simulink library "Storage_Type_3"  (R2018b)
settings: Solver=ode45  StartTime=0.0  StopTime=10.0  RelTol=1e-3  EnableMultiTasking=on
undefined symbols (not defined in the file): path_carnot
libraries: carnot x10
settings Model: Creator=bernd.hafner  LastModifiedBy=drhf
settings DataIOCC: LimitDataPoints=on  SaveFormat=Array  SignalLoggingSaveFormat=ModelDataLogs
settings OptimizationCC: ExpressionDepthLimit=2147483647  LifeSpan=inf
settings DebuggingCC: UnderspecifiedInitializationDetection=Classic  MergeDetectMultiDrivingBlocksExec=none  SolverPrmCheckMsg=warning  FcnCallInpInsideContextMsg=warning  StateNameClashWarn=warning  SFUnexpectedBacktrackingDiag=warning  SFNoUnconditionalDefaultTransitionDiag=warning  SFExecutionAtInitializationDiag=none
settings HardwareCC: ProdBitPerPointer=32  ProdBitPerSizeT=32  ProdBitPerPtrDiffT=32  ProdLargestAtomicFloat=None  ProdIntDivRoundTo=Undefined  ProdEndianess=Unspecified  ProdWordSize=32  ProdHWDeviceType=32-bit Generic
settings ModelReferenceCC: PropagateSignalLabelsOutOfModel=off
settings SFSimCC: SimUseLocalCustomCode=off
settings RTWCC: RTWUseLocalCustomCode=off
settings CodeAppCC: StateflowObjectComments=on
settings GRTTargetCC: TargetLangStandard=C89/C90 (ANSI)  CombineOutputUpdateFcns=off  GRTInterface=on
settings ConfigComp: CovMetricSettings=dw  CovHtmlReporting=on  CovSaveCumulativeToWorkspaceVar=on  CovSaveSingleToWorkspaceVar=on  CovExternalEMLEnable=off

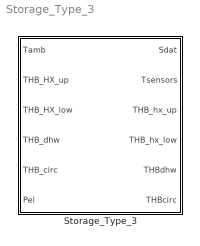
== system Storage_Type_3 ==
  Storage_Type_3 : Subsystem  mask(Storage for solar assisted hot water production){t0=[10:5:55], hgt=1.7684, stgtype=3, tini=[10 15 20 25 30 35 40 45 50 55], mpts=[1 2 3 4 5 6 7 8 9 10], PathName=fullfile(path_carnot('libsl'), 'Storage', 'Thermal', 'Storage_Type_3', 'parameter_set'), FileName='StorageType3_400_L.mat', userPath=off, userParam=off, uwall=1, ubot=1, utop=1, axcond=1, volume=0.5, dia=0.6, standing=standing cylinder, nodes=10, mpoints=10, Tsensor=[0.1 0.5 0.7], hx1inlet=0.8, hx1outlet=0.6, hx1dia=0.03, hx1uac=50, hx1uam=0.15, hx1uat=0.6, hx1_uat2=0, hx1dpqua=20, hx1dplin=20, hx2inlet=0.4, hx2outlet=0, hx2dia=0.03, hx2uac=100, hx2uam=0.15, hx2uat=0.6, hx2_uat2=0, hx2dplin=30, hx2dpqua=30, pipe1inlet=0, pipe1outlet=1, pipe1dia=0.03, pipe2inlet=0.6, pipe2outlet=1, pipe2dia=0.03, heater1start=0.6, heater1end=0.65}
      mask prompts: t0 "Initial temperature (vector or scalar) in °C"; hgt "Height of storage in m"; stgtype "Storage Type (0..5)"; tini "Start temperatures of nodes in °C"; mpts "Index to measured nodes"; PathName "Path"; FileName "Parameter set"; userPath "Edit path and name of parameter set"; userParam "User defined parameters"; uwall "Heat transfer coefficient to ambient [W/m²K]"; ubot "Heat transfer coefficient to ambient bottom [W/m²K]"; utop "Heat transfer coefficient to ambient top [W/m²K]"; axcond "Effective thermal conductivity [W/m/K]"; volume "Volume [m³]"; dia "Diameter [m]"; standing "Position"; nodes "Number of nodes"; mpoints "Number of node temperatures (for display)"; Tsensor "Temperature sensor position (0..1, 0 = bottom, 1 = top)"; hx1inlet "relative height of inlet"; hx1outlet "relative height of outlet"; hx1dia "Diameter of HX pipe [m]"; hx1uac "uac: heat transfer coefficient [W/K /(kg/s) /(°C)]"; hx1uam "uam: massflow dependent heat transfer [-]"; hx1uat "uat: temperature dependent heat transfer [-]"; hx1_uat2 "uat2: temperature difference dependent heat transfer [-]"; hx1dpqua "pressure drop quadratic in mdot [Pa*s²/kg²]"; hx1dplin "pressure drop linear in mdot [Pa*s/kg]"; hx2inlet "relative height of inlet"; hx2outlet "relative height of outlet"; hx2dia "Diameter of HX pipe [m]"; hx2uac "uac: heat transfer coefficient [W/K /(kg/s) /(°C)]"; hx2uam "uam: massflow dependent heat transfer [-]"; hx2uat "uat: temperature dependent heat transfer [-]"; hx2_uat2 "uat2: temperature difference dependent heat transfer [-]"; hx2dplin "pressure drop linear in mdot [Pa*s/kg]"; hx2dpqua "pressure drop quadratic in mdot [Pa*s²/kg²]"; pipe1inlet "relative height of inlet, range from 0 (= bottom) to 1 (= top)"; pipe1outlet "relative height of outlet, range from 0 (= bottom) to 1 (= top)"; pipe1dia "Diameter of pipe in m"; pipe2inlet "relative height of inlet, range from 0 (= bottom) to 1 (= top)"; pipe2outlet "relative height of outlet, range from 0 (= bottom) to 1 (= top)"; pipe2dia "Diameter of pipe in m"; heater1start "relative height start heating zone"; heater1end "relative height end heating zone"
      mask help:
      | Storage for hot water production (domestic hot water cylinder) with two heat exchangers.
      | The storage model has the following components (with their typical position):
      | - one solar heat exchanger (lower part)
      | - one backup heater heat exchanger (upper part)
      | - one pipe connection for the domestic hot water (total height)
      | - one pipe connection hot water circulation (upper part )
      mask init:
      | [ok, param] = CarnotCallbacks_StorageConf('SetParam',stgtype,gcbh,PathName,FileName);
      mask Help: web(fullfile(path_carnot('help'),'Storage_Type_N.html'),'-helpbrowser')
      mask TypeOptions hgt: HX_EN12977_1/hgt | HX_EN12977_2/hgt | Pipe_Connection_1/hgt | Pipe_Connection_2/hgt
      mask TypeOptions stgtype: CreateSdat/stgtype
      mask TypeOptions tini: sfun_storageTnodes/tini
      mask TypeOptions mpts: select_T/Indices
      mask Callback userPath: [ok, param] = CarnotCallbacks_StorageConf('UserEdit',3,gcbh);
      mask Callback userParam: [ok, param] = CarnotCallbacks_StorageConf('UserEdit',3,gcbh);
      mask TypeOptions uwall: sfun_storageTnodes/uloss
      mask TypeOptions ubot: sfun_storageTnodes/ubot
      mask TypeOptions utop: sfun_storageTnodes/utop
      mask TypeOptions axcond: sfun_storageTnodes/cond
      mask TypeOptions volume: sfun_storageTnodes/volume | CreateSdat/volume
      mask TypeOptions dia: sfun_storageTnodes/dia | Pipe_Connection_1/dstg | Pipe_Connection_2/dstg
      mask TypeOptions standing: sfun_storageTnodes/standing
      mask TypeOptions nodes: sfun_storageTnodes/nodes | select_T/InputPortWidth | HX_EN12977_1/nodes | HX_EN12977_2/nodes | Pipe_Connection_1/nodes | Pipe_Connection_2/nodes
      mask TypeOptions Tsensor: T_Sensor_Surface/pos
      mask TypeOptions hx1inlet: HX_EN12977_1/h_in
      mask TypeOptions hx1outlet: HX_EN12977_1/h_out
      mask TypeOptions hx1dia: HX_EN12977_1/dia
      mask TypeOptions hx1uac: HX_EN12977_1/ua0
      mask TypeOptions hx1uam: HX_EN12977_1/uam
      mask TypeOptions hx1uat: HX_EN12977_1/uat
      mask TypeOptions hx1_uat2: HX_EN12977_1/uat2
      mask TypeOptions hx1dpqua: HX_EN12977_1/dpqua
      mask TypeOptions hx1dplin: HX_EN12977_1/dplin
      mask TypeOptions hx2inlet: HX_EN12977_2/h_in
      mask TypeOptions hx2outlet: HX_EN12977_2/h_out
      mask TypeOptions hx2dia: HX_EN12977_2/dia
      mask TypeOptions hx2uac: HX_EN12977_2/ua0
      mask TypeOptions hx2uam: HX_EN12977_2/uam
      mask TypeOptions hx2uat: HX_EN12977_2/uat
      mask TypeOptions hx2_uat2: HX_EN12977_2/uat2
      mask TypeOptions hx2dplin: HX_EN12977_2/dplin
      mask TypeOptions hx2dpqua: HX_EN12977_2/dpqua
      mask TypeOptions pipe1inlet: Pipe_Connection_1/h_in
      mask TypeOptions pipe1outlet: Pipe_Connection_1/h_out
      mask TypeOptions pipe1dia: Pipe_Connection_1/dpipe
      mask TypeOptions pipe2inlet: Pipe_Connection_2/h_in
      mask TypeOptions pipe2outlet: Pipe_Connection_2/h_out
      mask TypeOptions pipe2dia: Pipe_Connection_2/dpipe
      mask TypeOptions heater1start: Electric_Heating_1/hin
      mask TypeOptions heater1end: Electric_Heating_1/hout
      mask DialogControl Container14 Prompt: Infos
      mask DialogControl ParameterGroupVar Prompt: Picking a parameter set
      mask DialogControl Control3 Prompt: Carnot public data
      mask DialogControl Control3 Callback: [ok, file] = CarnotCallbacks_StorageConf('GetFilename',3,gcbh,'public');
      mask DialogControl Control4 Prompt: Carnot internal data
      mask DialogControl Control4 Callback: [ok, file] = CarnotCallbacks_StorageConf('GetFilename',3,gcbh,'internal');
      mask DialogControl Control2 Prompt: Selected path
      mask DialogControl Control2 Callback: [ok, file] = CarnotCallbacks_StorageConf('GetFilename',3,gcbh,'selected');
      mask DialogControl Container4 Prompt: Parameter values
      mask DialogControl Container6 Prompt: Storage
      mask DialogControl Container8 Prompt: Connections
      mask DialogControl Container11 Prompt: Upper heat exchanger
      mask DialogControl Container13 Prompt: Lower heat exchanger
      mask DialogControl Container9 Prompt: Discharging pipe
      mask DialogControl Container12 Prompt: Circulation pipe
      mask DialogControl Container17 Prompt: Electric Heating
      mask DialogControl Container20 Prompt: Heater 1
      mask DialogControl Control6 Prompt: Save in Carnot internal data
      mask DialogControl Control6 Callback: [ok, param] = CarnotCallbacks_StorageConf('SaveFilename',3,gcbh,'internal','STG');
      mask DialogControl Control5 Prompt: Save in selected path
      mask DialogControl Control5 Callback: [ok, param] = CarnotCallbacks_StorageConf('SaveFilename',3,gcbh,'selected','STG');
      mask Display:
      | % user defined picture file
      | namestr = ['Storage_Type_', num2str(get_param(gcb,'stgtype'))];
      | picfile = fullfile(path_carnot('intlibsl'), 'Storage','Thermal', ...
      |     namestr,'parameter_set', [namestr, '.jpg']);
      | 
      | % show internal picture if defined
      | pic = false;
      | if  ~BlockIsInCarnotLibrary       % if not located in library
      |     if exist(picfile, 'file')
      |         image(imread(picfile), [0.25, 0, 0.45, 1])
      |         set_param(gcb, 'BackgroundColor', 'White')
      |         pic = true;
      |     end
      | end
      | 
      | % show public picture
      | if ~pic
      |     set_param(gcb, 'BackgroundColor', 'Red')
      |     plot([36,36,40,50,54,54,50,40,36]/90,[90,50,45,45,50,90,93,93,90]/100, ...
      |         [36,51,40,51,36]/90,[77,77,81,85,85]/100,[36,51,44,51,36]/90, ...
      |         [50,50,55,60,60]/100,...
      |         [36,50,50,36]/90,[75,75,74,74]/100,...
      |         [36,34,34,36]/90,[76.5,76.5,73,73]/100)
      | end

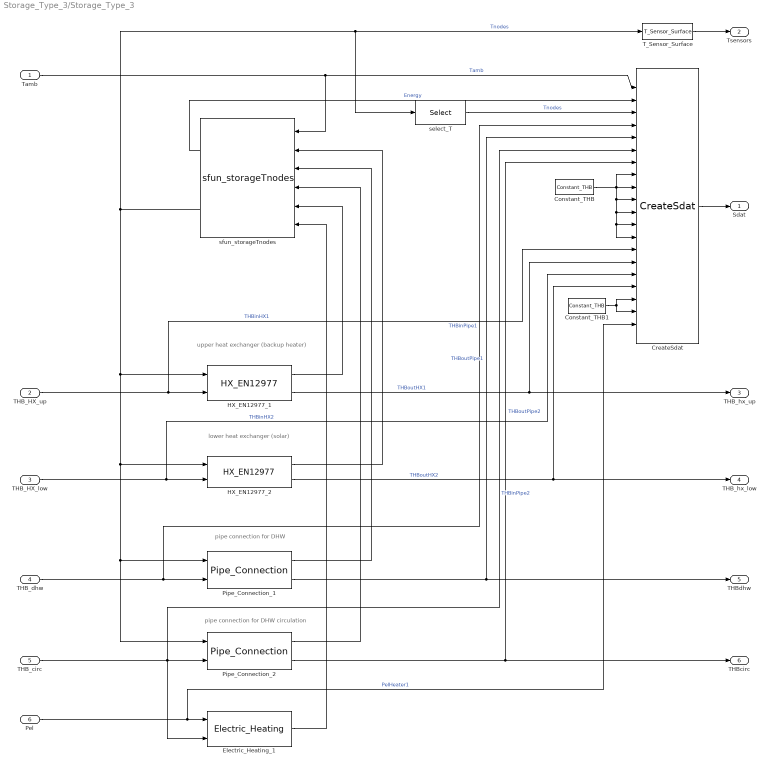
== system Storage_Type_3/Storage_Type_3 ==
  note: upper heat exchanger (backup heater)
  note: pipe connection for DHW
  note: pipe connection for DHW circulation
  note: lower heat exchanger (solar)
  Tamb : Inport
  THB_HX_up : Inport  Port=2
  THB_HX_low : Inport  Port=3
  THB_dhw : Inport  Port=4
  THB_circ : Inport  Port=5
  Pel : Inport  Port=6
  Constant_THB : carnot/Source/Simple/Constant_THB  t=20  mdot=0  p=1e5  mID=No Pressure Drop  fluid=Water  mix=0  mix2=0  mix3=0  dia=0.02  hgt=0
      settings: SourceProductName=Carnot
  Constant_THB1 : carnot/Source/Simple/Constant_THB  t=20  mdot=0  p=1e5  mID=No Pressure Drop  fluid=Water  mix=0  mix2=0  mix3=0  dia=0.02  hgt=0
      settings: SourceProductName=Carnot
  CreateSdat : carnot/Basic/Thermal_Models/CreateSdat  volume=volume  stgtype=stgtype
      settings: SourceProductName=Carnot
  Electric_Heating_1 : carnot/Storage/Thermal/Storage_Ports/Electric_Heating  hin=heater1start  hout=heater1end  nodes=nodes
      settings: SourceProductName=Carnot
  HX_EN12977_1 : carnot/Storage/Thermal/Storage_Ports/HX_EN12977  h_in=hx1inlet  h_out=hx1outlet  hgt=hgt  dia=hx1dia  height=-0.35368  ua0=hx1uac  uam=hx1uam  uat=hx1uat  uat2=hx1_uat2  dplin=hx1dplin  dpqua=hx1dpqua  nodes=nodes
      settings: SourceProductName=Carnot
  HX_EN12977_2 : carnot/Storage/Thermal/Storage_Ports/HX_EN12977  h_in=hx2inlet  h_out=hx2outlet  hgt=hgt  dia=hx2dia  height=-0.70736  ua0=hx2uac  uam=hx2uam  uat=hx2uat  uat2=hx2_uat2  dplin=hx2dplin  dpqua=hx2dpqua  nodes=nodes
      settings: SourceProductName=Carnot
  Pipe_Connection_1 : carnot/Storage/Thermal/Storage_Ports/Pipe_Connection  h_in=pipe1inlet  h_out=pipe1outlet  hgt=hgt  dpipe=pipe1dia  dstg=dia  height=1.7684  nodes=nodes
      settings: SourceProductName=Carnot
  Pipe_Connection_2 : carnot/Storage/Thermal/Storage_Ports/Pipe_Connection  h_in=pipe2inlet  h_out=pipe2outlet  hgt=hgt  dpipe=pipe2dia  dstg=dia  height=0.70736  nodes=nodes
      settings: SourceProductName=Carnot
  T_Sensor_Surface : carnot/Control/T_Sensor_Surface  pos=Tsensor  tdel=10  t0=mean(tini)
      settings: SourceProductName=Carnot
  select_T : Selector  InputPortWidth=nodes  IndexOptions=Index vector (dialog)  Indices=[1 2 3 4 5 6 7 8 9 10]  OutputSizes=1
  sfun_storageTnodes : carnot/Basic/Thermal_Models/sfun_storageTnodes  uloss=uwall  ubot=ubot  utop=utop  cond=axcond  volume=volume  dia=dia  standing=standing cylinder  tini=tini  nodes=nodes  nconnect=5  elimthermocline=2  condinvtc=1e5
      settings: SourceProductName=Carnot
  Sdat : Outport
  Tsensors : Outport  Port=2
  THB_hx_up : Outport  Port=3
  THB_hx_low : Outport  Port=4
  THBdhw : Outport  Port=5
  THBcirc : Outport  Port=6
  wires:
  Constant_THB/1 -> CreateSdat/9, CreateSdat/8, CreateSdat/13, CreateSdat/12, CreateSdat/11, CreateSdat/10
  Constant_THB1/1 -> CreateSdat/19, CreateSdat/18
  sfun_storageTnodes/1 -> CreateSdat/2  "Energy"
  HX_EN12977_1/1 -> sfun_storageTnodes/5
  Pipe_Connection_2/2 -> CreateSdat/7, THBcirc/1  "THBoutPipe2"
  Pipe_Connection_2/1 -> sfun_storageTnodes/4
  THB_circ/1 -> Electric_Heating_1/2, Pipe_Connection_2/2, CreateSdat/6  "THBinPipe2"
  Tamb/1 -> CreateSdat/1, sfun_storageTnodes/1  "Tamb"
  THB_HX_low/1 -> HX_EN12977_2/2, CreateSdat/16  "THBinHX2"
  HX_EN12977_2/2 -> THB_hx_low/1, CreateSdat/17  "THBoutHX2"
  HX_EN12977_2/1 -> sfun_storageTnodes/2
  select_T/1 -> CreateSdat/3  "Tnodes"
  sfun_storageTnodes/2 -> select_T/1, T_Sensor_Surface/1, HX_EN12977_1/1, HX_EN12977_2/1, Pipe_Connection_1/1, Pipe_Connection_2/1  "Tnodes"
  CreateSdat/1 -> Sdat/1
  THB_dhw/1 -> Pipe_Connection_1/2, CreateSdat/4  "THBinPipe1"
  Pipe_Connection_1/2 -> CreateSdat/5, THBdhw/1  "THBoutPipe1"
  Pipe_Connection_1/1 -> sfun_storageTnodes/3
  THB_HX_up/1 -> HX_EN12977_1/2, CreateSdat/14  "THBinHX1"
  HX_EN12977_1/2 -> THB_hx_up/1, CreateSdat/15  "THBoutHX1"
  T_Sensor_Surface/1 -> Tsensors/1
  Pel/1 -> Electric_Heating_1/1, CreateSdat/20  "PelHeater1"
  Electric_Heating_1/1 -> sfun_storageTnodes/6
